simulink model "V2x_blockset"  (Simulink 7.6)
settings: Solver=ode45  StartTime=0.0  StopTime=10.0  RelTol=1e-3
undefined symbols (not defined in the file or in its folder): intmax, Newton, Raphson
libraries: simulink x53
(part 2 of 3)

== system V2x_blockset/signs CAM generator/set CAM signals ==
  warning : Inport
  messageID : Inport  Port=2
  actorID : Inport  Port=3
  actorType : Inport  Port=4
  publicActorType : Inport  Port=5
  lightBarInUse : Inport  Port=6
  sireneInUse : Inport  Port=7
  velocity : Inport  Port=8
  acceleration : Inport  Port=9
  yawRate : Inport  Port=10
  turnAdvice : Inport  Port=11
  trafficLightPriority : Inport  Port=12
  GPS_lat : Inport  Port=13
  GPS_long : Inport  Port=14
  GPS_alt : Inport  Port=15
  rotZ : Inport  Port=16
  Mux : Mux  Inputs=16
  CAM_signals : Outport
  wires:
  warning/1 -> Mux/1
  messageID/1 -> Mux/2
  actorID/1 -> Mux/3
  actorType/1 -> Mux/4
  publicActorType/1 -> Mux/5
  lightBarInUse/1 -> Mux/6
  sireneInUse/1 -> Mux/7
  velocity/1 -> Mux/8
  acceleration/1 -> Mux/9
  yawRate/1 -> Mux/10
  turnAdvice/1 -> Mux/11
  trafficLightPriority/1 -> Mux/12
  GPS_lat/1 -> Mux/13
  GPS_long/1 -> Mux/14
  GPS_alt/1 -> Mux/15
  rotZ/1 -> Mux/16
  Mux/1 -> CAM_signals/1

== system V2x_blockset/vehicle CAM generator/CAM generation ==
  x [m] : Inport
  y [m] : Inport  Port=2
  z [m] : Inport  Port=3
  rotZ [deg] : Inport  Port=4
  velocity [m/s] : Inport  Port=5
  Enable : EnablePort  StatesWhenEnabling=reset  PropagateVarSize=During execution
  Add : Sum  Inputs=+-
  Data Store Memory : DataStoreMemory  DataStoreName=CAM_time
  Data Store Memory1 : DataStoreMemory  DataStoreName=CAM_velocity
  Data Store Memory2 : DataStoreMemory  DataStoreName=CAM_heading
  Data Store Memory3 : DataStoreMemory  DataStoreName=CAM_x
  Data Store Memory4 : DataStoreMemory  DataStoreName=CAM_y
  Data Store Memory5 : DataStoreMemory  DataStoreName=CAM_z
  Data Store Read : DataStoreRead  DataStoreName=CAM_time  SampleTime=0.01
  Digital Clock : DigitalClock  SampleTime=0.01
  Merge : Merge  Inputs=3
  if : If  IfExpression=u1 >= 1  ElseIfExpressions=u1 < 0.1
  maybe : Subsystem  TreatAsAtomicUnit=on
  no : Subsystem  TreatAsAtomicUnit=on
  yes : Subsystem  TreatAsAtomicUnit=on
  CAN generation signal : Outport  OutputWhenDisabled=reset  InitialOutput=0
  wires:
  Digital Clock/1 -> Add/1
  Data Store Read/1 -> Add/2
  Add/1 -> if/1
  if/1 -> yes/Action
  yes/1(Out1) -> Merge/1
  no/1(Out1) -> Merge/2
  if/2 -> no/Action
  if/3 -> maybe/Action
  Merge/1 -> CAN generation signal/1
  x [m]/1 -> maybe/1(x [m]), yes/1(x [m])
  y [m]/1 -> maybe/2(y [m]), yes/2(y [m])
  z [m]/1 -> maybe/3(z [m]), yes/3(z [m])
  rotZ [deg]/1 -> maybe/4(rotZ [deg]), yes/4(rotZ [deg])
  velocity [m/s]/1 -> maybe/5(velocity [m/s]), yes/5(velocity [m/s])
  maybe/1(Out1) -> Merge/3

== system V2x_blockset/vehicle CAM generator/Enabled Subsystem ==
  CAM_sig : Inport
  Enable : EnablePort  PropagateVarSize=During execution
  CAM_signals : Outport  OutputWhenDisabled=reset  InitialOutput=0
  wires:
  CAM_sig/1 -> CAM_signals/1

== system V2x_blockset/vehicle CAM generator/Subsystem ==
  In1 : Inport
  GPS_Noise_src : Inport  Port=2
  GPS Noise : Subsystem
  Sum2 : Sum  Inputs=|++
  Out1 : Outport
  wires:
  GPS Noise/1(GPS_Noise) -> Sum2/2
  In1/1 -> Sum2/1
  Sum2/1 -> Out1/1
  GPS_Noise_src/1 -> GPS Noise/1(GPS_Noise_src)

== system V2x_blockset/vehicle CAM generator/Subsystem1 ==
  In1 : Inport
  GPS_Noise_src : Inport  Port=2
  GPS Noise : Subsystem
  Sum2 : Sum  Inputs=|++
  Out1 : Outport
  wires:
  GPS_Noise_src/1 -> GPS Noise/1(GPS_Noise_src)
  Sum2/1 -> Out1/1
  In1/1 -> Sum2/1
  GPS Noise/1(GPS_Noise) -> Sum2/2

== system V2x_blockset/vehicle CAM generator/Subsystem2 ==
  In1 : Inport
  GPS_Noise_src : Inport  Port=2
  GPS Noise : Subsystem
  Sum2 : Sum  Inputs=|++
  Out1 : Outport
  wires:
  GPS Noise/1(GPS_Noise) -> Sum2/2
  In1/1 -> Sum2/1
  Sum2/1 -> Out1/1
  GPS_Noise_src/1 -> GPS Noise/1(GPS_Noise_src)

== system V2x_blockset/vehicle CAM generator/Subsystem3 ==
  In1 : Inport
  GPS_Noise_src : Inport  Port=2
  GPS Noise : Subsystem
  Sum2 : Sum  Inputs=|++
  Out1 : Outport
  wires:
  GPS_Noise_src/1 -> GPS Noise/1(GPS_Noise_src)
  Sum2/1 -> Out1/1
  In1/1 -> Sum2/1
  GPS Noise/1(GPS_Noise) -> Sum2/2

== system V2x_blockset/vehicle CAM generator/impulse generator ==
  CAM_time_step : Inport
  Add : Sum
  Compare To Zero : simulink/Logic and Bit Operations/Compare To Zero  SystemSampleTime=-1  relop=>  LogicOutDataTypeMode=boolean  ZeroCross=off
  Data Type Conversion : DataTypeConversion  OutDataTypeStr=boolean
  Detect Change : simulink/Logic and Bit Operations/Detect Change  SystemSampleTime=-1  vinit=0
  Digital Clock1 : DigitalClock  SampleTime=0.01
  Divide : Product  Inputs=*/
  Gain : Gain  Gain=pi
  Product : Product  RndMeth=Zero
  Trigonometric Function : Trigonometry
  constant : Constant
  experiment time step : Constant  Value=0.01  SampleTime=0
  enable : Outport
  wires:
  Digital Clock1/1 -> Product/1
  Gain/1 -> Product/2
  Trigonometric Function/1 -> Compare To Zero/1
  Compare To Zero/1 -> Detect Change/1
  Detect Change/1 -> Data Type Conversion/1
  Product/1 -> Add/1
  constant/1 -> Divide/1
  Divide/1 -> Gain/1
  Add/1 -> Trigonometric Function/1
  experiment time step/1 -> Add/2
  Data Type Conversion/1 -> enable/1
  CAM_time_step/1 -> Divide/2

== system V2x_blockset/vehicle CAM generator/impulse generator1 ==
  CAM_time_step : Inport
  Add : Sum
  Compare To Zero : simulink/Logic and Bit Operations/Compare To Zero  SystemSampleTime=-1  relop=>  LogicOutDataTypeMode=boolean  ZeroCross=off
  Data Type Conversion : DataTypeConversion  OutDataTypeStr=boolean
  Detect Change : simulink/Logic and Bit Operations/Detect Change  SystemSampleTime=-1  vinit=0
  Digital Clock1 : DigitalClock  SampleTime=0.01
  Divide : Product  Inputs=*/
  Gain : Gain  Gain=pi
  Product : Product  RndMeth=Zero
  Trigonometric Function : Trigonometry
  constant : Constant
  experiment time step : Constant  Value=0.01  SampleTime=0
  enable : Outport
  wires:
  CAM_time_step/1 -> Divide/2
  Data Type Conversion/1 -> enable/1
  experiment time step/1 -> Add/2
  Add/1 -> Trigonometric Function/1
  Divide/1 -> Gain/1
  constant/1 -> Divide/1
  Product/1 -> Add/1
  Detect Change/1 -> Data Type Conversion/1
  Compare To Zero/1 -> Detect Change/1
  Trigonometric Function/1 -> Compare To Zero/1
  Gain/1 -> Product/2
  Digital Clock1/1 -> Product/1

== system V2x_blockset/vehicle CAM generator/set CAM signals ==
  CAM generation signal : Inport
  warning : Inport  Port=2
  messageID : Inport  Port=3
  vehicleID : Inport  Port=4
  vehicleType : Inport  Port=5
  publicVehicleType : Inport  Port=6
  lightBarInUse : Inport  Port=7
  sireneInUse : Inport  Port=8
  velocity : Inport  Port=9
  acceleration : Inport  Port=10
  yawRate : Inport  Port=11
  turnAdvice : Inport  Port=12
  trafficLightPriority : Inport  Port=13
  GPS_lat : Inport  Port=14
  GPS_long : Inport  Port=15
  GPS_alt : Inport  Port=16
  rotZ : Inport  Port=17
  Mux : Mux  Inputs=16
  Switch : Switch  Criteria=u2 > Threshold  Threshold=0.5
  Unit Delay : UnitDelay  SampleTime=-1
  CAM_signals : Outport
  wires:
  warning/1 -> Mux/1
  messageID/1 -> Mux/2
  vehicleID/1 -> Mux/3
  vehicleType/1 -> Mux/4
  publicVehicleType/1 -> Mux/5
  lightBarInUse/1 -> Mux/6
  sireneInUse/1 -> Mux/7
  velocity/1 -> Mux/8
  acceleration/1 -> Mux/9
  yawRate/1 -> Mux/10
  turnAdvice/1 -> Mux/11
  trafficLightPriority/1 -> Mux/12
  GPS_lat/1 -> Mux/13
  GPS_long/1 -> Mux/14
  GPS_alt/1 -> Mux/15
  rotZ/1 -> Mux/16
  CAM generation signal/1 -> Switch/2
  Mux/1 -> Switch/1
  Switch/1 -> Unit Delay/1, CAM_signals/1
  Unit Delay/1 -> Switch/3

== system V2x_blockset/EEB/vehicle CAM generator/CAM delay ==
  in : Inport
  Tdelay : Inport  Port=2
  Bias : Bias  Bias=1
  Integer Delay{,1..9} (10 alike) : simulink/Discrete/Integer Delay  vinit=0.0  samptime=0.01  NumDelays=10
  Multiport Switch : MultiPortSwitch  Inputs=11  zeroidx=off
  Rounding Function : Rounding
  Saturation : Saturate  UpperLimit=11  LowerLimit=1
  out : Outport
  wires:
  Integer Delay9/1 -> Multiport Switch/12
  Saturation/1 -> Multiport Switch/1
  Bias/1 -> Saturation/1
  Rounding Function/1 -> Bias/1
  Tdelay/1 -> Rounding Function/1
  in/1 -> Integer Delay/1, Multiport Switch/2
  Integer Delay/1 -> Integer Delay1/1, Multiport Switch/3
  Integer Delay1/1 -> Integer Delay2/1, Multiport Switch/4
  Integer Delay2/1 -> Integer Delay3/1, Multiport Switch/5
  Integer Delay3/1 -> Integer Delay4/1, Multiport Switch/6
  Integer Delay4/1 -> Integer Delay5/1, Multiport Switch/7
  Integer Delay5/1 -> Integer Delay6/1, Multiport Switch/8
  Integer Delay6/1 -> Integer Delay7/1, Multiport Switch/9
  Integer Delay7/1 -> Integer Delay8/1, Multiport Switch/10
  Integer Delay8/1 -> Integer Delay9/1, Multiport Switch/11
  Multiport Switch/1 -> out/1

== system V2x_blockset/EEB/vehicle CAM generator/For Iterator Subsystem ==
  CAM_in : Inport
  Size : Inport  Port=2
  CAM_old : Inport  Port=3
  NoMM : Inport  Port=4
  tmp_in : Inport  Port=5
  Assignment : Assignment  NumberOfDimensions=2  IndexOptions=Assign all,Index vector (port)  Indices=-1,-1  OutputSizes=2,16
  Assignment1 : Assignment  NumberOfDimensions=2  IndexOptions=Assign all,Index vector (port)  Indices=-1,-1  OutputSizes=2,16
  Continuous signal : Stateflow chart  TreatAsAtomicUnit=on
  For Iterator : ForIterator  IterationSource=external
  Math Function{,1..3} (4 alike) : Math  Operator=transpose  SaturateOnIntegerOverflow=on
  Selector : Selector  NumberOfDimensions=2  InputPortWidth=3  IndexOptions=Select all,Index vector (dialog)  Indices=[1 3],1  OutputSizes=1,1
  CAM_o : Outport
  tmp_out : Outport  Port=2
  wires:
  For Iterator/1 -> Assignment/3, Assignment1/3, Continuous signal/3(i)
  CAM_in/1 -> Selector/1, Continuous signal/1(CAM), Math Function/1
  Size/1 -> For Iterator/1
  Assignment/1 -> Math Function3/1
  Continuous signal/1(CAM_o) -> Math Function1/1
  Math Function/1 -> Assignment/1
  Math Function1/1 -> Assignment/2
  Math Function3/1 -> CAM_o/1
  CAM_old/1 -> Continuous signal/2(CAM_old)
  NoMM/1 -> Continuous signal/4(NoMM)
  Continuous signal/2(tmp_out) -> Assignment1/2
  tmp_in/1 -> Continuous signal/5(tmp_in)
  Assignment1/1 -> tmp_out/1
  Selector/1 -> Math Function2/1
  Math Function2/1 -> Assignment1/1

== system V2x_blockset/GLOSA/vehicle CAM generator/CAM delay ==
  in : Inport
  Tdelay : Inport  Port=2
  Bias : Bias  Bias=1
  Integer Delay{,1..9} (10 alike) : simulink/Discrete/Integer Delay  vinit=0.0  samptime=0.01  NumDelays=10
  Multiport Switch : MultiPortSwitch  Inputs=11  zeroidx=off
  Rounding Function : Rounding
  Saturation : Saturate  UpperLimit=11  LowerLimit=1
  out : Outport
  wires:
  Integer Delay9/1 -> Multiport Switch/12
  Saturation/1 -> Multiport Switch/1
  Bias/1 -> Saturation/1
  Rounding Function/1 -> Bias/1
  Tdelay/1 -> Rounding Function/1
  in/1 -> Integer Delay/1, Multiport Switch/2
  Integer Delay/1 -> Integer Delay1/1, Multiport Switch/3
  Integer Delay1/1 -> Integer Delay2/1, Multiport Switch/4
  Integer Delay2/1 -> Integer Delay3/1, Multiport Switch/5
  Integer Delay3/1 -> Integer Delay4/1, Multiport Switch/6
  Integer Delay4/1 -> Integer Delay5/1, Multiport Switch/7
  Integer Delay5/1 -> Integer Delay6/1, Multiport Switch/8
  Integer Delay6/1 -> Integer Delay7/1, Multiport Switch/9
  Integer Delay7/1 -> Integer Delay8/1, Multiport Switch/10
  Integer Delay8/1 -> Integer Delay9/1, Multiport Switch/11
  Multiport Switch/1 -> out/1

== system V2x_blockset/GLOSA/vehicle CAM generator/For Iterator Subsystem ==
  CAM_in : Inport
  Size : Inport  Port=2
  CAM_old : Inport  Port=3
  NoMM : Inport  Port=4
  tmp_in : Inport  Port=5
  Assignment : Assignment  NumberOfDimensions=2  IndexOptions=Assign all,Index vector (port)  Indices=-1,-1  OutputSizes=2,16
  Assignment1 : Assignment  NumberOfDimensions=2  IndexOptions=Assign all,Index vector (port)  Indices=-1,-1  OutputSizes=2,16
  Continuous signal : Stateflow chart  TreatAsAtomicUnit=on
  For Iterator : ForIterator  IterationSource=external
  Math Function{,1..3} (4 alike) : Math  Operator=transpose  SaturateOnIntegerOverflow=on
  Selector : Selector  NumberOfDimensions=2  InputPortWidth=3  IndexOptions=Select all,Index vector (dialog)  Indices=[1 3],1  OutputSizes=1,1
  CAM_o : Outport
  tmp_out : Outport  Port=2
  wires:
  For Iterator/1 -> Assignment/3, Assignment1/3, Continuous signal/3(i)
  CAM_in/1 -> Selector/1, Continuous signal/1(CAM), Math Function/1
  Size/1 -> For Iterator/1
  Assignment/1 -> Math Function2/1
  Continuous signal/1(CAM_o) -> Math Function1/1
  Math Function/1 -> Assignment/1
  Math Function1/1 -> Assignment/2
  Math Function2/1 -> CAM_o/1
  CAM_old/1 -> Continuous signal/2(CAM_old)
  NoMM/1 -> Continuous signal/4(NoMM)
  Continuous signal/2(tmp_out) -> Assignment1/2
  tmp_in/1 -> Continuous signal/5(tmp_in)
  Assignment1/1 -> tmp_out/1
  Selector/1 -> Math Function3/1
  Math Function3/1 -> Assignment1/1

== system V2x_blockset/Traffic Controller/Intersection warning controller/Enabled Subsystem ==
  crossingType : Inport
  hostTurnAdvice : Inport  Port=2
  hostRotZ : Inport  Port=3
  host GPS lat [deg] : Inport  Port=4
  host GPS long [deg] : Inport  Port=5
  host GPS alt [m] : Inport  Port=6
  GPS_lat : Inport  Port=7
  GPS_long : Inport  Port=8
  GPS_alt : Inport  Port=9
  actorID : Inport  Port=10
  targetVelocity : Inport  Port=11
  turnAdvice : Inport  Port=12
  rotZ : Inport  Port=13
  actorType : Inport  Port=14
  crossing detection range : Inport  Port=15
  Enable : EnablePort  PropagateVarSize=During execution
  Intersection : Subsystem
  sort using ID : Subsystem
  warning left lane : Outport
  warning straight lane : Outport  Port=2
  warning right lane : Outport  Port=3
  wires:
  hostRotZ/1 -> Intersection/1(hostRotZ)
  hostTurnAdvice/1 -> Intersection/2(hostTurnAdvice)
  host GPS lat [deg]/1 -> Intersection/3(host GPS lat [deg])
  host GPS long [deg]/1 -> Intersection/4(host GPS long [deg])
  host GPS alt [m]/1 -> Intersection/5(host GPS alt [m])
  actorID/1 -> sort using ID/1(IDs)
  GPS_lat/1 -> sort using ID/2(in1)
  GPS_long/1 -> sort using ID/3(in2)
  GPS_alt/1 -> sort using ID/4(in3)
  targetVelocity/1 -> sort using ID/5(in4)
  turnAdvice/1 -> sort using ID/6(in5)
  rotZ/1 -> sort using ID/7(in6)
  actorType/1 -> sort using ID/8(in7)
  crossingType/1 -> sort using ID/9(in8)
  sort using ID/1(Out1) -> Intersection/6(GPS_lat)
  sort using ID/2(Out2) -> Intersection/7(GPS_long)
  sort using ID/3(Out3) -> Intersection/8(GPS_alt)
  sort using ID/4(Out4) -> Intersection/9(targetVelocity)
  sort using ID/5(Out5) -> Intersection/10(turnAdvice)
  sort using ID/6(Out6) -> Intersection/11(rotZ)
  sort using ID/7(Out7) -> Intersection/12(actorType)
  sort using ID/8(Out8) -> Intersection/13(crossingType)
  Intersection/1(warning left lane) -> warning left lane/1
  Intersection/2(warning straight lane) -> warning straight lane/1
  Intersection/3(warning right lane) -> warning right lane/1
  crossing detection range/1 -> Intersection/14(crossing detection range)

== system V2x_blockset/Traffic Controller/Road accident detection controller/Compute distance to road accident ==
  conditions : Inport
  host_GPS lat [deg] : Inport  Port=2
  host_GPS lat [deg]1 : Inport  Port=3
  host_GPS alt [m] : Inport  Port=4
  GPS lat [deg] : Inport  Port=5
  GPS long [deg] : Inport  Port=6
  GPS alt [deg] : Inport  Port=7
  Enable : EnablePort  ShowOutputPort=on
  If : If  IfExpression=u1
  If Action Subsystem : Subsystem  TreatAsAtomicUnit=on
  If Action Subsystem1 : Subsystem  TreatAsAtomicUnit=on
  Merge : Merge
  RA_warning : Outport  OutputWhenDisabled=reset  InitialOutput=0
  RA_distance : Outport  Port=2  OutputWhenDisabled=reset  InitialOutput=0
  wires:
  GPS alt [deg]/1 -> If Action Subsystem/4(GPS alt1)
  If/2 -> If Action Subsystem1/Action
  If Action Subsystem1/1(distance) -> Merge/2
  If Action Subsystem/1(distance) -> Merge/1
  GPS long [deg]/1 -> If Action Subsystem/3(GPS long1)
  GPS lat [deg]/1 -> If Action Subsystem/2(GPS lat1)
  If/1 -> If Action Subsystem/Action
  host_GPS lat [deg]1/1 -> If Action Subsystem/6(host_GPS_long)
  host_GPS lat [deg]/1 -> If Action Subsystem/5(host_GPS_lat)
  host_GPS alt [m]/1 -> If Action Subsystem/7(host_GPS_alt)
  Enable/1 -> If/1, RA_warning/1
  conditions/1 -> If Action Subsystem/1(conditions)
  Merge/1 -> RA_distance/1

== system V2x_blockset/Traffic Controller/Road accident detection controller/distance hold ==
  dist : Inport
  Constant : Constant  Value=0
  Discrete FIR Filter : DiscreteFir  NumCoeffs=0.1 * ones(1,10)
  Memory : Memory
  Switch : Switch  Criteria=u2 > Threshold
  Switch1 : Switch  Criteria=u2 ~= 0
  distance : Outport
  wires:
  dist/1 -> Switch/2, Switch/1, Discrete FIR Filter/1
  Switch/1 -> Memory/1, Switch1/1
  Memory/1 -> Switch/3
  Discrete FIR Filter/1 -> Switch1/2
  Constant/1 -> Switch1/3
  Switch1/1 -> distance/1

== system V2x_blockset/Traffic Controller/Road accident detection controller/warning hold ==
  warn : Inport
  Constant : Constant  Value=0
  Discrete FIR Filter : DiscreteFir  NumCoeffs=0.1 * ones(1,10)
  Memory : Memory
  Switch : Switch  Criteria=u2 > Threshold
  Switch1 : Switch  Criteria=u2 ~= 0
  warning : Outport
  wires:
  warn/1 -> Switch/2, Switch/1, Discrete FIR Filter/1
  Switch/1 -> Memory/1, Switch1/1
  Memory/1 -> Switch/3
  Discrete FIR Filter/1 -> Switch1/2
  Constant/1 -> Switch1/3
  Switch1/1 -> warning/1

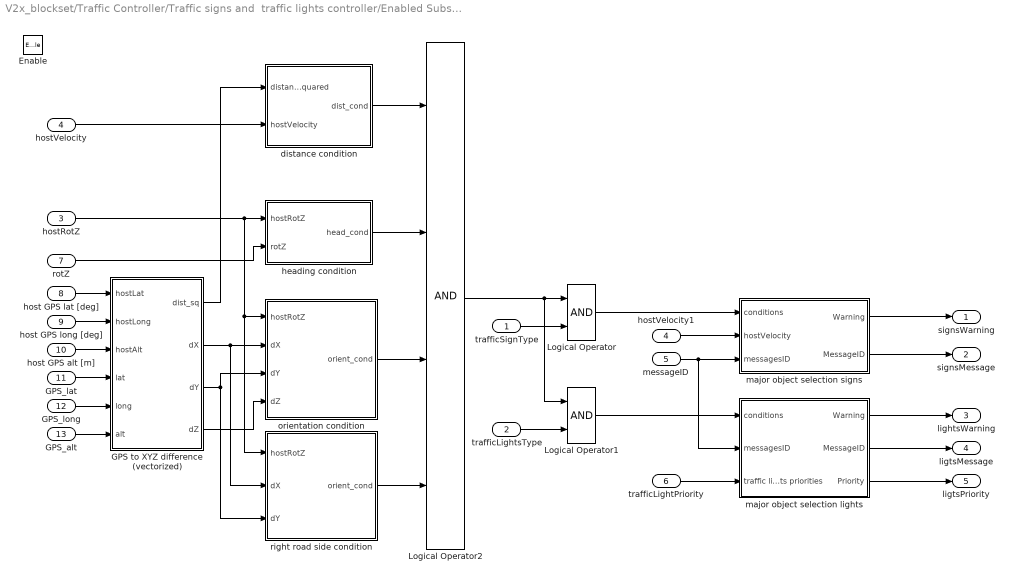
== system V2x_blockset/Traffic Controller/Traffic signs and  traffic lights controller/Enabled Subsystem ==
  trafficSignType : Inport
  trafficLightsType : Inport  Port=2
  hostRotZ : Inport  Port=3
  hostVelocity : Inport  Port=4
  messageID : Inport  Port=5
  trafficLightPriority : Inport  Port=6
  rotZ : Inport  Port=7
  host GPS lat [deg] : Inport  Port=8
  host GPS long [deg] : Inport  Port=9
  host GPS alt [m] : Inport  Port=10
  GPS_lat : Inport  Port=11
  GPS_long : Inport  Port=12
  GPS_alt : Inport  Port=13
  Enable : EnablePort  StatesWhenEnabling=reset  PropagateVarSize=During execution
  GPS to XYZ difference (vectorized) : Subsystem
  Logical Operator : Logic  AllPortsSameDT=off  OutDataTypeStr=boolean
  Logical Operator1 : Logic  AllPortsSameDT=off  OutDataTypeStr=boolean
  Logical Operator2 : Logic  Inputs=4  AllPortsSameDT=off  OutDataTypeStr=boolean
  distance condition : Subsystem
  heading condition : Subsystem
  hostVelocity1 : InportShadow  Port=4
  major object selection lights : Subsystem
  major object selection signs : Subsystem
  orientation condition : Subsystem
  right road side condition : Subsystem
  signsWarning : Outport
  signsMessage : Outport  Port=2  InitialOutput=0
  lightsWarning : Outport  Port=3
  ligtsMessage : Outport  Port=4  InitialOutput=0
  ligtsPriority : Outport  Port=5  InitialOutput=0
  wires:
  GPS to XYZ difference (vectorized)/3(dY) -> right road side condition/3(dY), orientation condition/3(dY)
  right road side condition/1(orient_cond) -> Logical Operator2/4
  GPS to XYZ difference (vectorized)/1(dist_sq) -> distance condition/1(distance_squared)
  GPS to XYZ difference (vectorized)/2(dX) -> orientation condition/2(dX), right road side condition/2(dX)
  GPS to XYZ difference (vectorized)/4(dZ) -> orientation condition/4(dZ)
  GPS_alt/1 -> GPS to XYZ difference (vectorized)/6(alt)
  orientation condition/1(orient_cond) -> Logical Operator2/3
  GPS_long/1 -> GPS to XYZ difference (vectorized)/5(long)
  GPS_lat/1 -> GPS to XYZ difference (vectorized)/4(lat)
  host GPS alt [m]/1 -> GPS to XYZ difference (vectorized)/3(hostAlt)
  host GPS long [deg]/1 -> GPS to XYZ difference (vectorized)/2(hostLong)
  host GPS lat [deg]/1 -> GPS to XYZ difference (vectorized)/1(hostLat)
  hostVelocity1/1 -> major object selection signs/2(hostVelocity)
  major object selection lights/3(Priority) -> ligtsPriority/1
  major object selection lights/2(MessageID) -> ligtsMessage/1
  major object selection lights/1(Warning) -> lightsWarning/1
  trafficLightPriority/1 -> major object selection lights/3(traffic lights priorities)
  Logical Operator1/1 -> major object selection lights/1(conditions)
  major object selection signs/2(MessageID) -> signsMessage/1
  major object selection signs/1(Warning) -> signsWarning/1
  messageID/1 -> major object selection lights/2(messagesID), major object selection signs/3(messagesID)
  Logical Operator/1 -> major object selection signs/1(conditions)
  trafficLightsType/1 -> Logical Operator1/2
  trafficSignType/1 -> Logical Operator/2
  Logical Operator2/1 -> Logical Operator1/1, Logical Operator/1
  heading condition/1(head_cond) -> Logical Operator2/2
  distance condition/1(dist_cond) -> Logical Operator2/1
  hostRotZ/1 -> orientation condition/1(hostRotZ), right road side condition/1(hostRotZ), heading condition/1(hostRotZ)
  hostVelocity/1 -> distance condition/2(hostVelocity)
  rotZ/1 -> heading condition/2(rotZ)

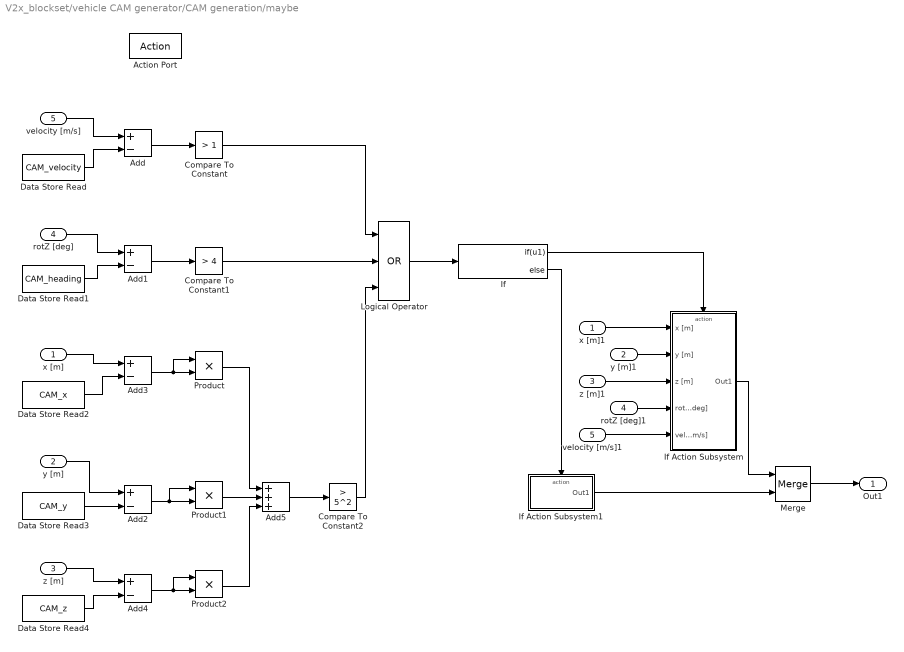
== system V2x_blockset/vehicle CAM generator/CAM generation/maybe ==
  x [m] : Inport
  y [m] : Inport  Port=2
  z [m] : Inport  Port=3
  rotZ [deg] : Inport  Port=4
  velocity [m/s] : Inport  Port=5
  Action Port : ActionPort  PropagateVarSize=During execution
  Add{,1..4} (5 alike) : Sum  Inputs=+-
  Add5 : Sum  Inputs=+++
  Compare To Constant : simulink/Logic and Bit Operations/Compare To Constant  SystemSampleTime=-1  relop=>  const=1  LogicOutDataTypeMode=boolean  ZeroCross=off
  Compare To Constant1 : simulink/Logic and Bit Operations/Compare To Constant  SystemSampleTime=-1  relop=>  const=4  LogicOutDataTypeMode=boolean  ZeroCross=off
  Compare To Constant2 : simulink/Logic and Bit Operations/Compare To Constant  SystemSampleTime=-1  relop=>  const=5^2  LogicOutDataTypeMode=boolean  ZeroCross=off
  Data Store Read : DataStoreRead  DataStoreName=CAM_velocity  SampleTime=0.01
  Data Store Read1 : DataStoreRead  DataStoreName=CAM_heading  SampleTime=0.01
  Data Store Read2 : DataStoreRead  DataStoreName=CAM_x  SampleTime=0.01
  Data Store Read3 : DataStoreRead  DataStoreName=CAM_y  SampleTime=0.01
  Data Store Read4 : DataStoreRead  DataStoreName=CAM_z  SampleTime=0.01
  If : If  IfExpression=u1
  If Action Subsystem : Subsystem  TreatAsAtomicUnit=on
  If Action Subsystem1 : Subsystem  TreatAsAtomicUnit=on
  Logical Operator : Logic  Operator=OR  Inputs=3  AllPortsSameDT=off  OutDataTypeStr=boolean
  Merge : Merge
  Product : Product  RndMeth=Zero
  Product1 : Product  RndMeth=Zero
  Product2 : Product  RndMeth=Zero
  rotZ [deg]1 : InportShadow  Port=4
  velocity [m/s]1 : InportShadow  Port=5
  x [m]1 : InportShadow  Port=1
  y [m]1 : InportShadow  Port=2
  z [m]1 : InportShadow  Port=3
  Out1 : Outport  OutputWhenDisabled=reset  InitialOutput=0
  wires:
  velocity [m/s]/1 -> Add/1
  Data Store Read/1 -> Add/2
  Add/1 -> Compare To Constant/1
  Add1/1 -> Compare To Constant1/1
  rotZ [deg]/1 -> Add1/1
  Data Store Read1/1 -> Add1/2
  x [m]/1 -> Add3/1
  Data Store Read2/1 -> Add3/2
  y [m]/1 -> Add2/1
  Data Store Read3/1 -> Add2/2
  z [m]/1 -> Add4/1
  Data Store Read4/1 -> Add4/2
  Add4/1 -> Product2/2, Product2/1
  Add2/1 -> Product1/2, Product1/1
  Add3/1 -> Product/2, Product/1
  Product/1 -> Add5/1
  Product1/1 -> Add5/2
  Product2/1 -> Add5/3
  Add5/1 -> Compare To Constant2/1
  Compare To Constant/1 -> Logical Operator/1
  Compare To Constant1/1 -> Logical Operator/2
  Compare To Constant2/1 -> Logical Operator/3
  Logical Operator/1 -> If/1
  If/1 -> If Action Subsystem/Action
  If/2 -> If Action Subsystem1/Action
  If Action Subsystem/1(Out1) -> Merge/1
  If Action Subsystem1/1(Out1) -> Merge/2
  Merge/1 -> Out1/1
  x [m]1/1 -> If Action Subsystem/1(x [m])
  y [m]1/1 -> If Action Subsystem/2(y [m])
  z [m]1/1 -> If Action Subsystem/3(z [m])
  rotZ [deg]1/1 -> If Action Subsystem/4(rotZ [deg])
  velocity [m/s]1/1 -> If Action Subsystem/5(velocity [m/s])

== system V2x_blockset/vehicle CAM generator/CAM generation/no ==
  Action Port : ActionPort  PropagateVarSize=During execution
  Constant : Constant  Value=0
  Out1 : Outport  OutputWhenDisabled=reset  InitialOutput=0
  wires:
  Constant/1 -> Out1/1

== system V2x_blockset/vehicle CAM generator/CAM generation/yes ==
  x [m] : Inport
  y [m] : Inport  Port=2
  z [m] : Inport  Port=3
  rotZ [deg] : Inport  Port=4
  velocity [m/s] : Inport  Port=5
  Action Port : ActionPort  PropagateVarSize=During execution
  Constant : Constant
  Data Store Write : DataStoreWrite  DataStoreName=CAM_velocity
  Data Store Write1 : DataStoreWrite  DataStoreName=CAM_heading
  Data Store Write2 : DataStoreWrite  DataStoreName=CAM_x
  Data Store Write3 : DataStoreWrite  DataStoreName=CAM_y
  Data Store Write4 : DataStoreWrite  DataStoreName=CAM_z
  Data Store Write5 : DataStoreWrite  DataStoreName=CAM_time
  Digital Clock1 : DigitalClock  SampleTime=0.01
  Out1 : Outport  OutputWhenDisabled=reset  InitialOutput=0
  wires:
  Constant/1 -> Out1/1
  velocity [m/s]/1 -> Data Store Write/1
  rotZ [deg]/1 -> Data Store Write1/1
  x [m]/1 -> Data Store Write2/1
  y [m]/1 -> Data Store Write3/1
  z [m]/1 -> Data Store Write4/1
  Digital Clock1/1 -> Data Store Write5/1

== system V2x_blockset/vehicle CAM generator/Subsystem/GPS Noise ==
  GPS_Noise_src : Inport
  Band-Limited White Noise1 : simulink/Sources/Band-Limited White Noise  SystemSampleTime=-1  Cov=1.7  Ts=0.01  seed=randi(intmax, 1)
  Constant : Constant  Value=1/(360*44)
  Product : Product  Inputs=3  RndMeth=Zero
  GPS_Noise : Outport
  wires:
  GPS_Noise_src/1 -> Product/1
  Band-Limited White Noise1/1 -> Product/2
  Constant/1 -> Product/3
  Product/1 -> GPS_Noise/1

== system V2x_blockset/vehicle CAM generator/Subsystem1/GPS Noise ==
  GPS_Noise_src : Inport
  Band-Limited White Noise1 : simulink/Sources/Band-Limited White Noise  SystemSampleTime=-1  Cov=1.7  Ts=0.01  seed=randi(intmax, 1)
  Constant : Constant  Value=1/(360*44)
  Product : Product  Inputs=3  RndMeth=Zero
  GPS_Noise : Outport
  wires:
  Product/1 -> GPS_Noise/1
  Constant/1 -> Product/3
  Band-Limited White Noise1/1 -> Product/2
  GPS_Noise_src/1 -> Product/1

== system V2x_blockset/vehicle CAM generator/Subsystem2/GPS Noise ==
  GPS_Noise_src : Inport
  Band-Limited White Noise1 : simulink/Sources/Band-Limited White Noise  SystemSampleTime=-1  Cov=1.7  Ts=0.01  seed=randi(intmax, 1)
  Constant : Constant  Value=1/(360*44)
  Product : Product  Inputs=3  RndMeth=Zero
  GPS_Noise : Outport
  wires:
  GPS_Noise_src/1 -> Product/1
  Band-Limited White Noise1/1 -> Product/2
  Constant/1 -> Product/3
  Product/1 -> GPS_Noise/1

== system V2x_blockset/vehicle CAM generator/Subsystem3/GPS Noise ==
  GPS_Noise_src : Inport
  Band-Limited White Noise1 : simulink/Sources/Band-Limited White Noise  SystemSampleTime=-1  Cov=1.7  Ts=0.01  seed=randi(intmax, 1)
  Constant : Constant  Value=1/(360*44)
  Product : Product  Inputs=3  RndMeth=Zero
  GPS_Noise : Outport
  wires:
  Product/1 -> GPS_Noise/1
  Constant/1 -> Product/3
  Band-Limited White Noise1/1 -> Product/2
  GPS_Noise_src/1 -> Product/1

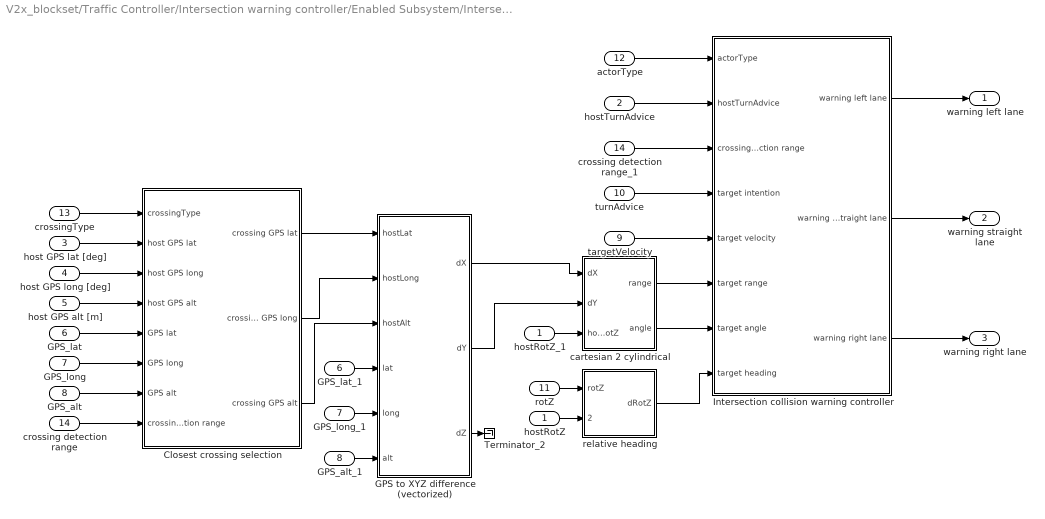
== system V2x_blockset/Traffic Controller/Intersection warning controller/Enabled Subsystem/Intersection ==
  hostRotZ : Inport
  hostTurnAdvice : Inport  Port=2
  host GPS lat [deg] : Inport  Port=3
  host GPS long [deg] : Inport  Port=4
  host GPS alt [m] : Inport  Port=5
  GPS_lat : Inport  Port=6
  GPS_long : Inport  Port=7
  GPS_alt : Inport  Port=8
  targetVelocity : Inport  Port=9
  turnAdvice : Inport  Port=10
  rotZ : Inport  Port=11
  actorType : Inport  Port=12
  crossingType : Inport  Port=13
  crossing detection range : Inport  Port=14
  Closest crossing selection : Subsystem
  GPS to XYZ difference (vectorized) : Subsystem
  GPS_alt_1 : InportShadow  Port=8
  GPS_lat_1 : InportShadow  Port=6
  GPS_long_1 : InportShadow  Port=7
  Intersection collision warning controller : Subsystem
  Terminator_2 : Terminator
  cartesian 2 cylindrical : Subsystem
  crossing detection range_1 : InportShadow  Port=14
  hostRotZ_1 : InportShadow  Port=1
  relative heading : Subsystem
  warning left lane : Outport
  warning straight lane : Outport  Port=2
  warning right lane : Outport  Port=3
  wires:
  host GPS lat [deg]/1 -> Closest crossing selection/2(host GPS lat)
  host GPS long [deg]/1 -> Closest crossing selection/3(host GPS long)
  host GPS alt [m]/1 -> Closest crossing selection/4(host GPS alt)
  Closest crossing selection/1(crossing GPS lat) -> GPS to XYZ difference (vectorized)/1(hostLat)
  Closest crossing selection/2(crossing GPS long) -> GPS to XYZ difference (vectorized)/2(hostLong)
  Closest crossing selection/3(crossing GPS alt) -> GPS to XYZ difference (vectorized)/3(hostAlt)
  crossing detection range/1 -> Closest crossing selection/8(crossing detection range)
  crossing detection range_1/1 -> Intersection collision warning controller/3(crossing detection range)
  hostRotZ/1 -> relative heading/2(hostRotZ)
  hostTurnAdvice/1 -> Intersection collision warning controller/2(hostTurnAdvice)
  cartesian 2 cylindrical/1(range) -> Intersection collision warning controller/6(target range)
  relative heading/1(dRotZ) -> Intersection collision warning controller/8(target heading)
  Intersection collision warning controller/1(warning left lane) -> warning left lane/1
  Intersection collision warning controller/2(warning straight lane) -> warning straight lane/1
  Intersection collision warning controller/3(warning right lane) -> warning right lane/1
  GPS to XYZ difference (vectorized)/1(dX) -> cartesian 2 cylindrical/1(dX)
  GPS to XYZ difference (vectorized)/2(dY) -> cartesian 2 cylindrical/2(dY)
  GPS_lat/1 -> Closest crossing selection/5(GPS lat)
  GPS_long/1 -> Closest crossing selection/6(GPS long)
  GPS_alt/1 -> Closest crossing selection/7(GPS alt)
  crossingType/1 -> Closest crossing selection/1(crossingType)
  rotZ/1 -> relative heading/1(rotZ)
  GPS_lat_1/1 -> GPS to XYZ difference (vectorized)/4(lat)
  GPS_long_1/1 -> GPS to XYZ difference (vectorized)/5(long)
  GPS_alt_1/1 -> GPS to XYZ difference (vectorized)/6(alt)
  turnAdvice/1 -> Intersection collision warning controller/4(target intention)
  targetVelocity/1 -> Intersection collision warning controller/5(target velocity)
  actorType/1 -> Intersection collision warning controller/1(actorType)
  GPS to XYZ difference (vectorized)/3(dZ) -> Terminator_2/1
  hostRotZ_1/1 -> cartesian 2 cylindrical/3(hostRotZ)
  cartesian 2 cylindrical/2(angle) -> Intersection collision warning controller/7(target angle)

== system V2x_blockset/Traffic Controller/Intersection warning controller/Enabled Subsystem/sort using ID ==
  IDs : Inport
  in1 : Inport  Port=2
  in2 : Inport  Port=3
  in3 : Inport  Port=4
  in4 : Inport  Port=5
  in5 : Inport  Port=6
  in6 : Inport  Port=7
  in7 : Inport  Port=8
  in8 : Inport  Port=9
  Embedded MATLAB Function : Stateflow chart  TreatAsAtomicUnit=on
  Selector{1..8} (8 alike) : Selector  IndexOptions=Index vector (port)  Indices=[1 3]  OutputSizes=1
  Out1 : Outport
  Out2 : Outport  Port=2
  Out3 : Outport  Port=3
  Out4 : Outport  Port=4
  Out5 : Outport  Port=5
  Out6 : Outport  Port=6
  Out7 : Outport  Port=7
  Out8 : Outport  Port=8
  wires:
  Embedded MATLAB Function/1(y) -> Selector7/2, Selector8/2, Selector6/2, Selector5/2, Selector4/2, Selector3/2, Selector2/2, Selector1/2
  IDs/1 -> Embedded MATLAB Function/1(ids)
  in7/1 -> Selector7/1
  in6/1 -> Selector6/1
  Selector7/1 -> Out7/1
  Selector6/1 -> Out6/1
  in5/1 -> Selector5/1
  in4/1 -> Selector4/1
  in3/1 -> Selector3/1
  in2/1 -> Selector2/1
  Selector5/1 -> Out5/1
  Selector4/1 -> Out4/1
  Selector3/1 -> Out3/1
  Selector2/1 -> Out2/1
  Selector1/1 -> Out1/1
  in1/1 -> Selector1/1
  in8/1 -> Selector8/1
  Selector8/1 -> Out8/1

== system V2x_blockset/Traffic Controller/Road accident detection controller/Compute distance to road accident/If Action Subsystem ==
  conditions : Inport
  GPS lat1 : Inport  Port=2
  GPS long1 : Inport  Port=3
  GPS alt1 : Inport  Port=4
  host_GPS_lat : Inport  Port=5
  host_GPS_long : Inport  Port=6
  host_GPS_alt : Inport  Port=7
  Action Port : ActionPort  PropagateVarSize=During execution
  GPS to distance : Subsystem
  Product7 : Product  RndMeth=Zero
  Product8 : Product  RndMeth=Zero
  Product9 : Product  RndMeth=Zero
  Sum6 : Sum  Inputs=+
  Sum7 : Sum  Inputs=+
  Sum8 : Sum  Inputs=+
  distance : Outport  InitialOutput=0
  wires:
  conditions/1 -> Product7/1, Product9/1, Product8/1
  GPS lat1/1 -> Product7/2
  GPS long1/1 -> Product8/2
  GPS alt1/1 -> Product9/2
  Product7/1 -> Sum6/1
  Product8/1 -> Sum7/1
  Product9/1 -> Sum8/1
  Sum6/1 -> GPS to distance/4(lat)
  Sum7/1 -> GPS to distance/5(long)
  Sum8/1 -> GPS to distance/6(alt)
  host_GPS_lat/1 -> GPS to distance/1(hostLat)
  host_GPS_long/1 -> GPS to distance/2(hostLong)
  host_GPS_alt/1 -> GPS to distance/3(hostAlt)
  GPS to distance/1(dist) -> distance/1

== system V2x_blockset/Traffic Controller/Road accident detection controller/Compute distance to road accident/If Action Subsystem1 ==
  Action Port : ActionPort  PropagateVarSize=During execution
  Constant : Constant  Value=0
  distance : Outport  InitialOutput=0
  wires:
  Constant/1 -> distance/1

== system V2x_blockset/Traffic Controller/Traffic signs and  traffic lights controller/Enabled Subsystem/GPS to XYZ difference (vectorized) ==
  hostLat : Inport
  hostLong : Inport  Port=2
  hostAlt : Inport  Port=3
  lat : Inport  Port=4
  long : Inport  Port=5
  alt : Inport  Port=6
  Add : Sum  Inputs=+-
  Add1 : Sum  Inputs=+-
  Add2 : Sum  Inputs=+-
  Add3 : Sum  Inputs=+++
  Product{,1..4} (5 alike) : Product  RndMeth=Zero
  d2r : Gain  Gain=pi/180
  d2r1 : Gain  Gain=pi/180
  mean Earth radius (latitudal) : Constant  Value=6335439.8775
  mean Earth radius (longitudal) : Constant  Value=6378137.55
  dist_sq : Outport
  dX : Outport  Port=2
  dY : Outport  Port=3
  dZ : Outport  Port=4
  wires:
  Add3/1 -> dist_sq/1
  Product4/1 -> Add3/3
  Product3/1 -> Add3/2
  Product/1 -> Add3/1
  Add2/1 -> Product4/1, Product4/2, dZ/1
  Product1/1 -> Product3/2, Product3/1, dX/1
  Product2/1 -> Product/2, Product/1, dY/1
  mean Earth radius (latitudal)/1 -> Product2/2
  mean Earth radius (longitudal)/1 -> Product1/2
  d2r1/1 -> Product1/1
  d2r/1 -> Product2/1
  Add1/1 -> d2r1/1
  Add/1 -> d2r/1
  hostAlt/1 -> Add2/2
  alt/1 -> Add2/1
  hostLong/1 -> Add1/2
  long/1 -> Add1/1
  hostLat/1 -> Add/2
  lat/1 -> Add/1

== system V2x_blockset/Traffic Controller/Traffic signs and  traffic lights controller/Enabled Subsystem/distance condition ==
  distance_squared : Inport
  hostVelocity : Inport  Port=2
  If : If  IfExpression=u1 ~= 0
  If Action Subsystem : Subsystem  TreatAsAtomicUnit=on
  If Action Subsystem1 : Subsystem  TreatAsAtomicUnit=on
  Merge : Merge
  Product3 : Product  RndMeth=Zero
  Product4 : Product  RndMeth=Zero
  Relational Operator1 : RelationalOperator  Operator=<  OutDataTypeStr=boolean
  headway time : Constant  Value=3
  dist_cond : Outport
  wires:
  Product3/1 -> If Action Subsystem1/1(headway time), Relational Operator1/2
  distance_squared/1 -> If Action Subsystem1/2(d2), If Action Subsystem/1(d2)
  Relational Operator1/1 -> dist_cond/1
  Merge/1 -> Relational Operator1/1
  If Action Subsystem1/1(t2) -> Merge/2
  If Action Subsystem/1(t2) -> Merge/1
  Product4/1 -> If Action Subsystem/2(v2)
  If/2 -> If Action Subsystem1/Action
  If/1 -> If Action Subsystem/Action
  hostVelocity/1 -> Product4/2, Product4/1, If/1
  headway time/1 -> Product3/1, Product3/2

== system V2x_blockset/Traffic Controller/Traffic signs and  traffic lights controller/Enabled Subsystem/heading condition ==
  hostRotZ : Inport
  rotZ : Inport  Port=2
  Abs : Abs
  Add : Sum  Inputs=+-
  Add1 : Sum  Inputs=-+
  Bias : Bias  Bias=180
  Constant : Constant  Value=360
  Constant1 : Constant  Value=360
  Logical Operator : Logic  Operator=OR  AllPortsSameDT=off  OutDataTypeStr=boolean
  Math Function : Math  Operator=mod  SaturateOnIntegerOverflow=on
  Relational Operator : RelationalOperator  Operator=<  OutDataTypeStr=boolean
  Relational Operator1 : RelationalOperator  Operator=>  OutDataTypeStr=boolean
  heading difference : Constant  Value=45
  head_cond : Outport
  wires:
  Logical Operator/1 -> head_cond/1
  Relational Operator1/1 -> Logical Operator/2
  Relational Operator/1 -> Logical Operator/1
  Constant1/1 -> Add1/2
  Add1/1 -> Relational Operator1/2
  heading difference/1 -> Add1/1, Relational Operator/2
  Abs/1 -> Relational Operator1/1, Relational Operator/1
  Math Function/1 -> Abs/1
  hostRotZ/1 -> Add/2
  rotZ/1 -> Add/1
  Bias/1 -> Math Function/1
  Constant/1 -> Math Function/2
  Add/1 -> Bias/1

== system V2x_blockset/Traffic Controller/Traffic signs and  traffic lights controller/Enabled Subsystem/major object selection lights ==
  conditions : Inport
  messagesID : Inport  Port=2
  traffic lights priorities : Inport  Port=3
  If : If  IfExpression=u1
  If Action Subsystem : Subsystem  TreatAsAtomicUnit=on
  If Action Subsystem1 : Subsystem  TreatAsAtomicUnit=on
  Logical Operator1 : Logic  Operator=OR  Inputs=1  AllPortsSameDT=off  OutDataTypeStr=boolean
  Merge : Merge
  Merge2 : Merge
  Traffic Lights Warning : Subsystem
  Warning : Outport
  MessageID : Outport  Port=2
  Priority : Outport  Port=3
  wires:
  Traffic Lights Warning/1(Warning) -> Warning/1
  Merge/1 -> Traffic Lights Warning/1(trafficLightPriority), Priority/1
  Merge2/1 -> MessageID/1
  If Action Subsystem/2(Priority) -> Merge/1
  If Action Subsystem/1(Message) -> Merge2/1
  If Action Subsystem1/1(Message) -> Merge2/2
  If Action Subsystem1/2(Priority) -> Merge/2
  traffic lights priorities/1 -> If Action Subsystem/3(traffic lights priorities)
  messagesID/1 -> If Action Subsystem/2(messagesID)
  conditions/1 -> If Action Subsystem/1(cond), Logical Operator1/1
  If/2 -> If Action Subsystem1/Action
  If/1 -> If Action Subsystem/Action
  Logical Operator1/1 -> If/1

== system V2x_blockset/Traffic Controller/Traffic signs and  traffic lights controller/Enabled Subsystem/major object selection signs ==
  conditions : Inport
  hostVelocity : Inport  Port=2
  messagesID : Inport  Port=3
  If : If  IfExpression=u1
  If Action Subsystem : Subsystem  TreatAsAtomicUnit=on
  If Action Subsystem1 : Subsystem  TreatAsAtomicUnit=on
  Logical Operator1 : Logic  Operator=OR  Inputs=1  AllPortsSameDT=off  OutDataTypeStr=boolean
  Merge : Merge
  Merge1 : Merge
  Warning : Outport
  MessageID : Outport  Port=2
  wires:
  hostVelocity/1 -> If Action Subsystem/3(hostVelocity)
  Merge/1 -> MessageID/1
  Merge1/1 -> Warning/1
  If Action Subsystem1/1(Warning) -> Merge1/2
  If Action Subsystem/1(Warning) -> Merge1/1
  If Action Subsystem/2(Message) -> Merge/1
  If Action Subsystem1/2(Message) -> Merge/2
  messagesID/1 -> If Action Subsystem/2(messagesID)
  conditions/1 -> If Action Subsystem/1(cond), Logical Operator1/1
  If/2 -> If Action Subsystem1/Action
  If/1 -> If Action Subsystem/Action
  Logical Operator1/1 -> If/1

== system V2x_blockset/Traffic Controller/Traffic signs and  traffic lights controller/Enabled Subsystem/orientation condition ==
  hostRotZ : Inport
  dX : Inport  Port=2
  dY : Inport  Port=3
  dZ : Inport  Port=4
  Abs : Abs
  Gain : Gain  Gain=pi/180
  Relational Operator : RelationalOperator  Operator=<  OutDataTypeStr=boolean
  Terminator : Terminator
  Trigonometric Function : Trigonometry  Operator=atan2
  d2r : Gain  Gain=pi/180
  orientation limit : Constant  Value=45
  to local reference system : Subsystem
  orient_cond : Outport
  wires:
  to local reference system/2(dx) -> Trigonometric Function/2
  to local reference system/1(dy) -> Trigonometric Function/1
  dY/1 -> to local reference system/3(dY)
  dX/1 -> to local reference system/2(dX)
  Gain/1 -> to local reference system/1(rotZ)
  hostRotZ/1 -> Gain/1
  Trigonometric Function/1 -> Abs/1
  Relational Operator/1 -> orient_cond/1
  d2r/1 -> Relational Operator/2
  Abs/1 -> Relational Operator/1
  orientation limit/1 -> d2r/1
  dZ/1 -> Terminator/1

== system V2x_blockset/Traffic Controller/Traffic signs and  traffic lights controller/Enabled Subsystem/right road side condition ==
  hostRotZ : Inport
  dX : Inport  Port=2
  dY : Inport  Port=3
  Compare To Zero : simulink/Logic and Bit Operations/Compare To Zero  SystemSampleTime=-1  relop=<  LogicOutDataTypeMode=boolean
  Gain : Gain  Gain=pi/180
  to local reference system : Subsystem
  orient_cond : Outport
  wires:
  Compare To Zero/1 -> orient_cond/1
  hostRotZ/1 -> Gain/1
  Gain/1 -> to local reference system/1(rotZ)
  dX/1 -> to local reference system/2(dX)
  dY/1 -> to local reference system/3(dY)
  to local reference system/1(dy) -> Compare To Zero/1

== system V2x_blockset/vehicle CAM generator/CAM generation/maybe/If Action Subsystem ==
  x [m] : Inport
  y [m] : Inport  Port=2
  z [m] : Inport  Port=3
  rotZ [deg] : Inport  Port=4
  velocity [m/s] : Inport  Port=5
  Action Port : ActionPort  PropagateVarSize=During execution
  Constant : Constant
  Data Store Write : DataStoreWrite  DataStoreName=CAM_velocity
  Data Store Write1 : DataStoreWrite  DataStoreName=CAM_heading
  Data Store Write2 : DataStoreWrite  DataStoreName=CAM_x
  Data Store Write3 : DataStoreWrite  DataStoreName=CAM_y
  Data Store Write4 : DataStoreWrite  DataStoreName=CAM_z
  Data Store Write5 : DataStoreWrite  DataStoreName=CAM_time
  Digital Clock1 : DigitalClock  SampleTime=0.01
  Out1 : Outport  InitialOutput=0
  wires:
  Constant/1 -> Out1/1
  velocity [m/s]/1 -> Data Store Write/1
  rotZ [deg]/1 -> Data Store Write1/1
  x [m]/1 -> Data Store Write2/1
  y [m]/1 -> Data Store Write3/1
  z [m]/1 -> Data Store Write4/1
  Digital Clock1/1 -> Data Store Write5/1

== system V2x_blockset/vehicle CAM generator/CAM generation/maybe/If Action Subsystem1 ==
  Action Port : ActionPort  PropagateVarSize=During execution
  Constant : Constant  Value=0
  Out1 : Outport  InitialOutput=0
  wires:
  Constant/1 -> Out1/1

== system V2x_blockset/Traffic Controller/Intersection warning controller/Enabled Subsystem/Intersection/Closest crossing selection ==
  crossingType : Inport
  host GPS lat : Inport  Port=2
  host GPS long : Inport  Port=3
  host GPS alt : Inport  Port=4
  GPS lat : Inport  Port=5
  GPS long : Inport  Port=6
  GPS alt : Inport  Port=7
  crossing detection range : Inport  Port=8
  GPS alt1 : InportShadow  Port=7
  GPS lat1 : InportShadow  Port=5
  GPS long1 : InportShadow  Port=6
  GPS to XYZ difference (vectorized) : Subsystem
  If : If  NumInputs=2  IfExpression=u1 ~= u2
  If Action Subsystem : Subsystem  TreatAsAtomicUnit=on
  If Action Subsystem1 : Subsystem  TreatAsAtomicUnit=on
  Logical Operator : Logic  AllPortsSameDT=off  OutDataTypeStr=boolean
  Merge : Merge
  Merge1 : Merge
  Merge2 : Merge
  MinMax : MinMax
  Product : Product  RndMeth=Zero
  Relational Operator : RelationalOperator  Operator=<  OutDataTypeStr=boolean
  Switch : Switch  Criteria=u2 > Threshold
  crossing GPS lat : Outport
  crossing GPS long : Outport  Port=2
  crossing GPS alt : Outport  Port=3
  wires:
  GPS to XYZ difference (vectorized)/1(dist_sq) -> Relational Operator/1, Switch/1, If Action Subsystem/2(dist_sq)
  crossing detection range/1 -> Product/2, Product/1
  Product/1 -> Relational Operator/2, Switch/3, If/2
  Relational Operator/1 -> Logical Operator/1
  crossingType/1 -> Logical Operator/2
  Logical Operator/1 -> Switch/2
  Switch/1 -> MinMax/1
  MinMax/1 -> If Action Subsystem/1(min), If/1
  host GPS lat/1 -> GPS to XYZ difference (vectorized)/1(hostLat)
  host GPS long/1 -> GPS to XYZ difference (vectorized)/2(hostLong)
  host GPS alt/1 -> GPS to XYZ difference (vectorized)/3(hostAlt)
  GPS lat/1 -> GPS to XYZ difference (vectorized)/4(lat)
  GPS long/1 -> GPS to XYZ difference (vectorized)/5(long)
  GPS alt/1 -> GPS to XYZ difference (vectorized)/6(alt)
  If/1 -> If Action Subsystem/Action
  If/2 -> If Action Subsystem1/Action
  GPS lat1/1 -> If Action Subsystem/3(GPS lat1)
  GPS long1/1 -> If Action Subsystem/4(GPS long1)
  GPS alt1/1 -> If Action Subsystem/5(GPS alt1)
  If Action Subsystem/1(GPS lat) -> Merge/1
  If Action Subsystem/2(GPS long) -> Merge2/1
  If Action Subsystem/3(GPS alt) -> Merge1/1
  If Action Subsystem1/1(GPS lat) -> Merge/2
  If Action Subsystem1/2(GPS long) -> Merge2/2
  If Action Subsystem1/3(GPS alt) -> Merge1/2
  Merge2/1 -> crossing GPS long/1
  Merge/1 -> crossing GPS lat/1
  Merge1/1 -> crossing GPS alt/1

== system V2x_blockset/Traffic Controller/Intersection warning controller/Enabled Subsystem/Intersection/GPS to XYZ difference (vectorized) ==
  hostLat : Inport
  hostLong : Inport  Port=2
  hostAlt : Inport  Port=3
  lat : Inport  Port=4
  long : Inport  Port=5
  alt : Inport  Port=6
  Add : Sum  Inputs=+-
  Add1 : Sum  Inputs=+-
  Add2 : Sum  Inputs=+-
  Product1 : Product  RndMeth=Zero
  Product2 : Product  RndMeth=Zero
  d2r : Gain  Gain=pi/180
  d2r1 : Gain  Gain=pi/180
  mean Earth radius (latitudal) : Constant  Value=6335439.8775
  mean Earth radius (longitudal) : Constant  Value=6378137.55
  dX : Outport
  dY : Outport  Port=2
  dZ : Outport  Port=3
  wires:
  lat/1 -> Add/1
  hostLat/1 -> Add/2
  long/1 -> Add1/1
  hostLong/1 -> Add1/2
  alt/1 -> Add2/1
  hostAlt/1 -> Add2/2
  Add/1 -> d2r/1
  Add1/1 -> d2r1/1
  d2r/1 -> Product2/1
  d2r1/1 -> Product1/1
  mean Earth radius (longitudal)/1 -> Product1/2
  mean Earth radius (latitudal)/1 -> Product2/2
  Product2/1 -> dY/1
  Product1/1 -> dX/1
  Add2/1 -> dZ/1

== system V2x_blockset/Traffic Controller/Intersection warning controller/Enabled Subsystem/Intersection/Intersection collision warning controller ==
  actorType : Inport
  hostTurnAdvice : Inport  Port=2
  crossing detection range : Inport  Port=3
  target intention : Inport  Port=4
  target velocity : Inport  Port=5
  target range : Inport  Port=6
  target angle : Inport  Port=7
  target heading : Inport  Port=8
  For Each Subsystem : Subsystem  TreatAsAtomicUnit=on
  Logical Operator : Logic  Operator=OR  Inputs=1  AllPortsSameDT=off  OutDataTypeStr=boolean
  Logical Operator1 : Logic  Operator=OR  Inputs=1  AllPortsSameDT=off  OutDataTypeStr=boolean
  Logical Operator2 : Logic  Operator=OR  Inputs=1  AllPortsSameDT=off  OutDataTypeStr=boolean
  host intention translation : Subsystem
  warning left lane : Outport
  warning straight lane : Outport  Port=2
  warning right lane : Outport  Port=3
  wires:
  hostTurnAdvice/1 -> host intention translation/1(host intention)
  For Each Subsystem/1(warning left lane) -> Logical Operator/1
  For Each Subsystem/2(warning straight lane) -> Logical Operator1/1
  For Each Subsystem/3(warning right lane) -> Logical Operator2/1
  actorType/1 -> For Each Subsystem/1(actorType)
  host intention translation/1(WM) -> For Each Subsystem/2(WM)
  crossing detection range/1 -> For Each Subsystem/3(Rcross)
  target range/1 -> For Each Subsystem/4(target range)
  target angle/1 -> For Each Subsystem/5(target angle)
  target intention/1 -> For Each Subsystem/6(target intention)
  target heading/1 -> For Each Subsystem/7(target heading)
  Logical Operator/1 -> warning left lane/1
  Logical Operator1/1 -> warning straight lane/1
  Logical Operator2/1 -> warning right lane/1
  target velocity/1 -> For Each Subsystem/8(targetVelocity)

== system V2x_blockset/Traffic Controller/Intersection warning controller/Enabled Subsystem/Intersection/cartesian 2 cylindrical ==
  dX : Inport
  dY : Inport  Port=2
  hostRotZ : Inport  Port=3
  Add : Sum  Inputs=+-
  Complex to Magnitude-Angle1 : ComplexToMagnitudeAngle
  Real-Imag to Complex1 : RealImagToComplex
  r2d : Gain  Gain=180/pi
  range : Outport
  angle : Outport  Port=2
  wires:
  Real-Imag to Complex1/1 -> Complex to Magnitude-Angle1/1
  dX/1 -> Real-Imag to Complex1/1
  Complex to Magnitude-Angle1/1 -> range/1  "range"
  dY/1 -> Real-Imag to Complex1/2
  Complex to Magnitude-Angle1/2 -> r2d/1  "angle"
  r2d/1 -> Add/1
  hostRotZ/1 -> Add/2
  Add/1 -> angle/1

== system V2x_blockset/Traffic Controller/Intersection warning controller/Enabled Subsystem/Intersection/relative heading ==
  rotZ : Inport
  hostRotZ : Inport  Port=2
  Add : Sum  Inputs=+-
  Constant : Constant  Value=360
  Math Function : Math  Operator=mod  SaturateOnIntegerOverflow=on
  dRotZ : Outport
  wires:
  Constant/1 -> Math Function/2
  rotZ/1 -> Add/1
  hostRotZ/1 -> Add/2
  Add/1 -> Math Function/1
  Math Function/1 -> dRotZ/1

== system V2x_blockset/Traffic Controller/Road accident detection controller/Compute distance to road accident/If Action Subsystem/GPS to distance ==
  hostLat : Inport
  hostLong : Inport  Port=2
  hostAlt : Inport  Port=3
  lat : Inport  Port=4
  long : Inport  Port=5
  alt : Inport  Port=6
  Add : Sum  Inputs=+-
  Add1 : Sum  Inputs=+-
  Add2 : Sum  Inputs=+-
  Add3 : Sum  Inputs=+++
  Product{,1..4} (5 alike) : Product  RndMeth=Zero
  Sqrt : Sqrt  AlgorithmType=Newton-Raphson  SaturateOnIntegerOverflow=on
  d2r : Gain  Gain=pi/180
  d2r1 : Gain  Gain=pi/180
  mean Earth radius (latitudal) : Constant  Value=6335439.8775
  mean Earth radius (longitudal) : Constant  Value=6378137.55
  dist : Outport
  wires:
  lat/1 -> Add/1
  hostLat/1 -> Add/2
  long/1 -> Add1/1
  hostLong/1 -> Add1/2
  alt/1 -> Add2/1
  hostAlt/1 -> Add2/2
  Add/1 -> d2r/1
  Add1/1 -> d2r1/1
  d2r/1 -> Product2/1
  d2r1/1 -> Product1/1
  mean Earth radius (longitudal)/1 -> Product1/2
  mean Earth radius (latitudal)/1 -> Product2/2
  Product2/1 -> Product/1, Product/2
  Product1/1 -> Product3/1, Product3/2
  Add2/1 -> Product4/2, Product4/1
  Product/1 -> Add3/1
  Product3/1 -> Add3/2
  Product4/1 -> Add3/3
  Add3/1 -> Sqrt/1
  Sqrt/1 -> dist/1

== system V2x_blockset/Traffic Controller/Traffic signs and  traffic lights controller/Enabled Subsystem/distance condition/If Action Subsystem ==
  d2 : Inport
  v2 : Inport  Port=2
  Action Port : ActionPort  PropagateVarSize=During execution
  Divide : Product  Inputs=*/
  t2 : Outport
  wires:
  Divide/1 -> t2/1
  v2/1 -> Divide/2
  d2/1 -> Divide/1
